simulink model "FOCandPMSM_plant"  (R2022b)
settings: Solver=FixedStepAuto  StartTime=0.0  StopTime=0.25  RelTol=1e-3  EnableMultiTasking=on
PreLoadFcn:
  | Ts = 1e-4;
  | Tcpu = 50e-6; %Controller sample time
  | 
  | % PMSM parameters
  | PM = 0.03; % Permanent magnet flux linkage
  | Ld = 2e-4;  % d-axis inductance
  | Lq = 2e-4;  % q-axis inductance
  | L0 = 2e-4;  % 0-axis inductance
  | Rs = 0.013; % Stator resistance
  | N = 6; % Number of pole pairs
  | J = 0.2; % Moment of inertia
  | 
  | % encoder parameters
  | numSlits = 2000; % number of slits
  | pulseSigOffset = 0; % index pulse signal offset
  | shaftInitPos = 0; % motor shaft initial position
  | 
  | % DAC parameters
  | gain = 0.1;
  | bias = 0;
  | 
  | % circuit parameters
  | Vdc = 48;
  | 
  | % real-time parameters
  | ts_FPGA_clk = 5e-9;
  | ts_FPGA_mdl = 1e-6;
  | 
  | % Real-time processor or embedded controller
  | RTorTTL = 1; % 1: Real-time processor,    0: embedded controller
  | 
  | % sample times
  | f_base = 200e6;
  | PWM_frequency = 20e3;
  | ts_FPGA_clk = 1/f_base;
  | ts_FPGA_mdl =1e-6;
values from neighbouring files (symbols this model uses):
  inverter = mcb_updateInverterParameters(pmsm,inverter,target)    [embedded_sim_codegen_data.m]
  pmsm = mcb_SetPMSMMotorParameters('Teknic2310P')    [embedded_sim_codegen_data.m]
  PU_System = mcb_SetPUSystem(pmsm,inverter)    [embedded_sim_codegen_data.m]
  SpeedRef = 1    [PMSM_HIL_Param.m]
  T_cpu = T_pwm    (= 5e-05)    [embedded_sim_codegen_data.m]
  Tsw = 1/f_sw    [PMSM_HIL_Param.m]
libraries: simulink x5, hdlsllib x3, mcbhdlplantlib x2, slrtencoderlib x2, slrtresolverlib x2, mcbpositiondecoderlib x2, slrthdlutillib x1, slrt2levelinverterlib x1, mcbcontrolslib x1
settings Model: Creator=chrisz  LastModifiedBy=chrisz
settings SolverCC: AutoInsertRateTranBlk=on
settings OptimizationCC: BlockReduction=off  ConditionallyExecuteInputs=off  DefaultParameterBehavior=Inlined
settings DebuggingCC: AlgebraicLoopMsg=error  SingleTaskRateTransMsg=error
settings HardwareCC: ProdBitPerPointer=32  ProdBitPerSizeT=32  ProdBitPerPtrDiffT=32  ProdLargestAtomicFloat=None  ProdIntDivRoundTo=Undefined  ProdEndianess=Unspecified  ProdWordSize=32  ProdHWDeviceType=ASIC/FPGA->ASIC/FPGA  TargetBitPerPointer=64  TargetBitPerSizeT=64  TargetBitPerPtrDiffT=64  TargetLongLongMode=on  TargetIntDivRoundTo=Zero  TargetEndianess=LittleEndian  TargetWordSize=64  TargetHWDeviceType=Custom Processor->MATLAB Host Computer  ProdEqTarget=off
settings ModelReferenceCC: EnableRefExpFcnMdlSchedulingChecks=on

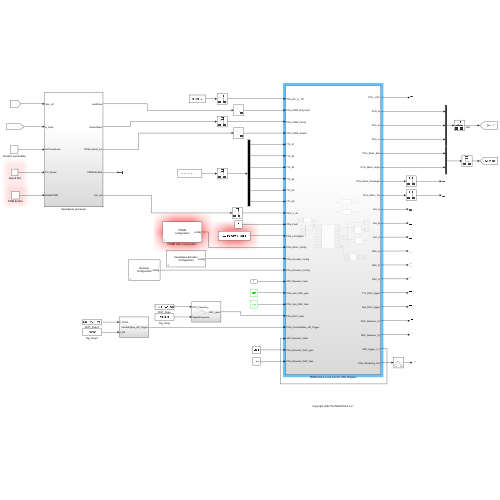
[thumbnail: Simulink's stored preview of the top-level diagram]
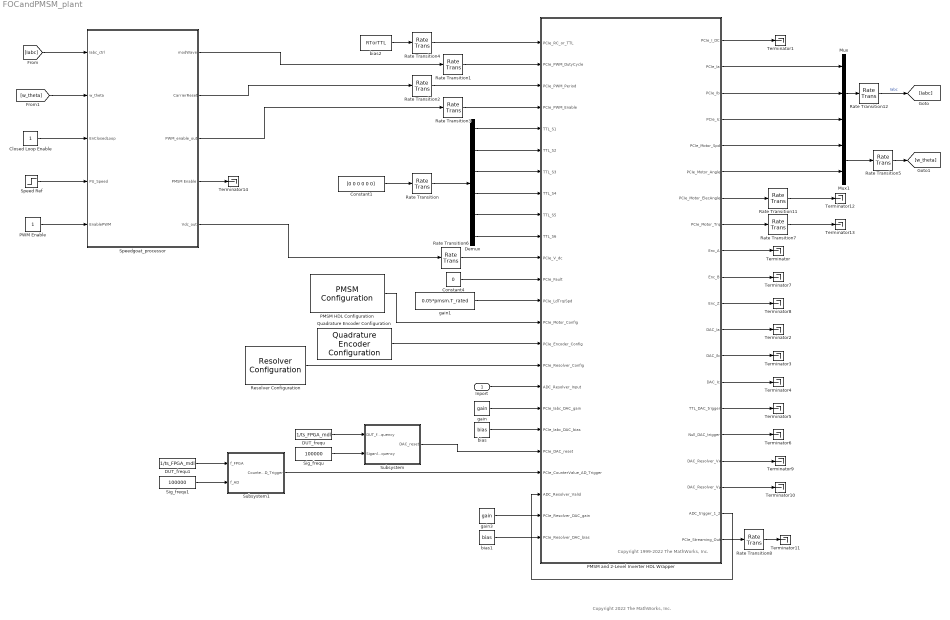
== system FOCandPMSM_plant ==
  note: Copyright 1999-2022 The MathWorks, Inc.
  note: Copyright 2022 The MathWorks, Inc.
  Inport : Inport  OutDataTypeStr=int16
  Closed Loop Enable : Constant  OutDataTypeStr=Inherit: Inherit via back propagation  SampleTime=-1
  Constant1 : Constant  Value=[0 0 0 0 0 0]  OutDataTypeStr=boolean  SampleTime=-1
  Constant4 : Constant  Value=0  OutDataTypeStr=uint32  SampleTime=ts_FPGA_mdl
  DUT_frequ : Constant  Value=1/ts_FPGA_mdl  SampleTime=ts_FPGA_mdl
  DUT_frequ1 : Constant  Value=1/ts_FPGA_mdl  SampleTime=ts_FPGA_mdl
  Demux : Demux  Outputs=6
  Mux : Mux  Inputs=3
  Mux1 : Mux  Inputs=2
  PMSM HDL Configuration : mcbhdlplantlib/PMSM Configuration  portConfig=Torque  Trq_N_mode=0  Ts=ts_FPGA_mdl  Pp=pmsm.p  Rs=pmsm.Rs  Ld=pmsm.Ld  Lq=pmsm.Lq  lambda_pm=pmsm.FluxPM  J=pmsm.J  B=0  f=0
      settings: LibrarySourceBlock=mcbhdllib/Electrical Systems/Motors/PMSM Configuration
  PMSM and 2-Level Inverter HDL Wrapper : Subsystem
  PWM Enable : Constant  OutDataTypeStr=Inherit: Inherit via back propagation  SampleTime=T_cpu
  Quadrature Encoder Configuration : slrtencoderlib/Quadrature Encoder Configuration  NPulses=2000  zOffset=0  Ts=ts_FPGA_mdl
  Rate Transition : RateTransition  OutPortSampleTime=ts_FPGA_clk
  Rate Transition{1..4,6} (5 alike) : RateTransition  OutPortSampleTime=ts_FPGA_mdl
  Rate Transition{5,7..8,11..12} (5 alike) : RateTransition  OutPortSampleTime=Tcpu
  Resolver Configuration : slrtresolverlib/Resolver Configuration  Ts=ts_FPGA_mdl  R=0.5  N=1  ADCrefV=5  ADCbits=16  totalADCCounts=65536
  Sig_frequ : Constant  Value=100000  VectorParams1D=off  SampleTime=ts_FPGA_mdl
  Sig_frequ1 : Constant  Value=100000  VectorParams1D=off  SampleTime=ts_FPGA_mdl
  Speed Ref : Step  Time=0.25  Before=1500/PU_System.N_base  After=SpeedRef  OutDataTypeStr=dataType  SampleTime=T_cpu
  Speedgoat_processor : Subsystem
  Subsystem : Subsystem
  Subsystem1 : Subsystem
  Terminator{,1..14} (15 alike) : Terminator
  bias : Constant  Value=bias  OutDataTypeStr=single  SampleTime=ts_FPGA_mdl
  bias1 : Constant  Value=bias  OutDataTypeStr=single  SampleTime=ts_FPGA_mdl
  bias2 : Constant  Value=RTorTTL  OutDataTypeStr=single  SampleTime=ts_FPGA_mdl
  gain : Constant  Value=gain  OutDataTypeStr=single  SampleTime=ts_FPGA_mdl
  gain1 : Constant  Value=0.05*pmsm.T_rated  OutDataTypeStr=single  SampleTime=ts_FPGA_mdl
  gain3 : Constant  Value=gain  OutDataTypeStr=single  SampleTime=ts_FPGA_mdl
  wires:
  PMSM and 2-Level Inverter HDL Wrapper/9(Enc_A) -> Terminator/1
  Rate Transition7/1 -> Terminator13/1
  PMSM and 2-Level Inverter HDL Wrapper/12(DAC_Ia) -> Terminator2/1
  PMSM and 2-Level Inverter HDL Wrapper/1(PCIe_I_DC) -> Terminator1/1
  PMSM and 2-Level Inverter HDL Wrapper/10(Enc_B) -> Terminator7/1
  PMSM and 2-Level Inverter HDL Wrapper/14(DAC_Ic) -> Terminator4/1
  PMSM and 2-Level Inverter HDL Wrapper/15(TTL_DAC_trigger) -> Terminator5/1
  PMSM and 2-Level Inverter HDL Wrapper/13(DAC_Ib) -> Terminator3/1
  PMSM and 2-Level Inverter HDL Wrapper/16(Null_DAC_trigger) -> Terminator6/1
  PMSM and 2-Level Inverter HDL Wrapper/5(PCIe_Motor_Spd) -> Mux1/1
  PMSM and 2-Level Inverter HDL Wrapper/6(PCIe_Motor_Angle) -> Mux1/2
  PMSM and 2-Level Inverter HDL Wrapper/8(PCIe_Motor_Trq) -> Rate Transition7/1
  PMSM and 2-Level Inverter HDL Wrapper/11(Enc_Z) -> Terminator8/1
  PMSM and 2-Level Inverter HDL Wrapper/17(DAC_Resolver_Vx) -> Terminator9/1
  PMSM and 2-Level Inverter HDL Wrapper/18(DAC_Resolver_Vy) -> Terminator10/1
  Rate Transition11/1 -> Terminator12/1
  PMSM and 2-Level Inverter HDL Wrapper/7(PCIe_Motor_ElecAngle) -> Rate Transition11/1
  Speedgoat_processor/4(PMSM Enable) -> Terminator14/1
  Demux/4 -> PMSM and 2-Level Inverter HDL Wrapper/8(TTL_S4)
  gain3/1 -> PMSM and 2-Level Inverter HDL Wrapper/23(PCIe_Resolver_DAC_gain)
  Subsystem/1(DAC_reset) -> PMSM and 2-Level Inverter HDL Wrapper/20(PCIe_DAC_reset)
  Rate Transition1/1 -> PMSM and 2-Level Inverter HDL Wrapper/2(PCIe_PWM_DutyCycle)
  Demux/2 -> PMSM and 2-Level Inverter HDL Wrapper/6(TTL_S2)
  Subsystem1/1(CounterValue_AD_Trigger) -> PMSM and 2-Level Inverter HDL Wrapper/21(PCIe_CounterValue_AD_Trigger)
  Demux/1 -> PMSM and 2-Level Inverter HDL Wrapper/5(TTL_S1)
  bias/1 -> PMSM and 2-Level Inverter HDL Wrapper/19(PCIe_Iabc_DAC_bias)
  Rate Transition4/1 -> PMSM and 2-Level Inverter HDL Wrapper/1(PCIe_RC_or_TTL)
  bias1/1 -> PMSM and 2-Level Inverter HDL Wrapper/24(PCIe_Resolver_DAC_bias)
  gain/1 -> PMSM and 2-Level Inverter HDL Wrapper/18(PCIe_Iabc_DAC_gain)
  Constant4/1 -> PMSM and 2-Level Inverter HDL Wrapper/12(PCIe_Fault)
  Rate Transition3/1 -> PMSM and 2-Level Inverter HDL Wrapper/4(PCIe_PWM_Enable)
  Rate Transition2/1 -> PMSM and 2-Level Inverter HDL Wrapper/3(PCIe_PWM_Period)
  Demux/3 -> PMSM and 2-Level Inverter HDL Wrapper/7(TTL_S3)
  PMSM HDL Configuration/1 -> PMSM and 2-Level Inverter HDL Wrapper/14(PCIe_Motor_Config)
  gain1/1 -> PMSM and 2-Level Inverter HDL Wrapper/13(PCIe_LdTrq/Spd)
  Resolver Configuration/1 -> PMSM and 2-Level Inverter HDL Wrapper/16(PCIe_Resolver_Config)
  PWM Enable/1 -> Speedgoat_processor/5(EnablePWM)
  Inport/1 -> PMSM and 2-Level Inverter HDL Wrapper/17(ADC_Resolver_Input)
  Speedgoat_processor/3(PWM_enable_out) -> Rate Transition3/1
  [Iabc] -> Speedgoat_processor/1(Iabc_ctrl)
  DUT_frequ1/1 -> Subsystem1/1(f_FPGA)
  DUT_frequ/1 -> Subsystem/1(DUT_frequency)
  Speed Ref/1 -> Speedgoat_processor/4(PU_Speed)
  Speedgoat_processor/2(CarrierReset) -> Rate Transition2/1
  bias2/1 -> Rate Transition4/1
  Closed Loop Enable/1 -> Speedgoat_processor/3(EnClosedLoop)
  Sig_frequ1/1 -> Subsystem1/2(f_AD)
  Sig_frequ/1 -> Subsystem/2(SiganlFrequency)
  Speedgoat_processor/1(modWave) -> Rate Transition1/1
  Constant1/1 -> Rate Transition/1
  Demux/6 -> PMSM and 2-Level Inverter HDL Wrapper/10(TTL_S6)
  Quadrature Encoder Configuration/1 -> PMSM and 2-Level Inverter HDL Wrapper/15(PCIe_Encoder_Config)
  Demux/5 -> PMSM and 2-Level Inverter HDL Wrapper/9(TTL_S5)
  [w_theta] -> Speedgoat_processor/2(w_theta)
  Rate Transition/1 -> Demux/1
  PMSM and 2-Level Inverter HDL Wrapper/19(ADC_trigger_1_2) -> PMSM and 2-Level Inverter HDL Wrapper/22(ADC_Resolver_Valid)
  Mux/1 -> Rate Transition12/1
  Rate Transition5/1 -> [w_theta]
  Mux1/1 -> Rate Transition5/1
  Speedgoat_processor/5(Vdc_out) -> Rate Transition6/1
  Rate Transition6/1 -> PMSM and 2-Level Inverter HDL Wrapper/11(PCIe_V_dc)
  PMSM and 2-Level Inverter HDL Wrapper/2(PCIe_Ia) -> Mux/1
  PMSM and 2-Level Inverter HDL Wrapper/3(PCIe_Ib) -> Mux/2
  PMSM and 2-Level Inverter HDL Wrapper/4(PCIe_Ic) -> Mux/3
  Rate Transition12/1 -> [Iabc]  "Iabc"
  PMSM and 2-Level Inverter HDL Wrapper/20(PCIe_Streaming_Out) -> Rate Transition8/1
  Rate Transition8/1 -> Terminator11/1

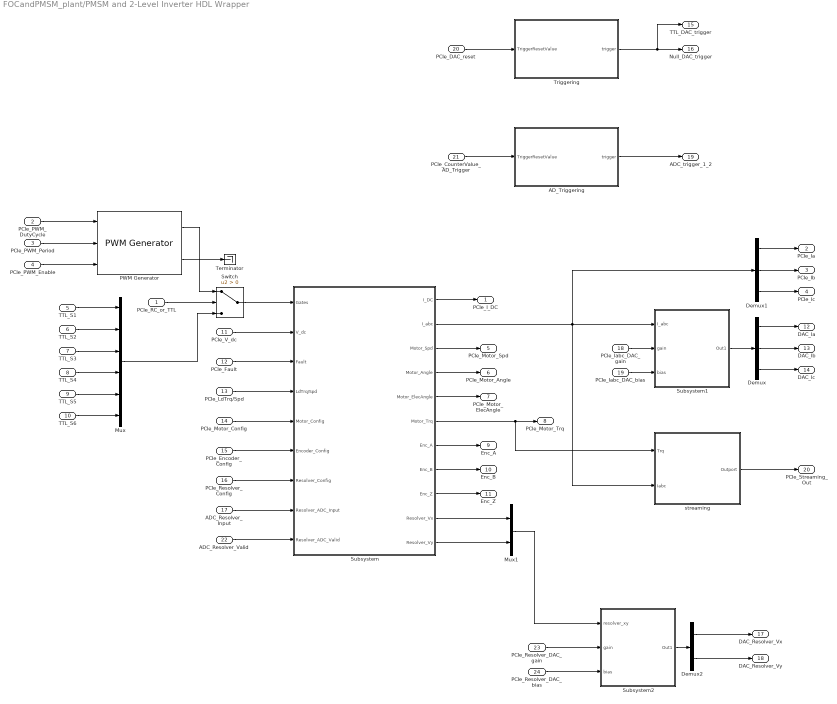
== system FOCandPMSM_plant/PMSM and 2-Level Inverter HDL Wrapper ==
  PCIe_RC_or_TTL : Inport
  PCIe_PWM_DutyCycle : Inport  Port=2
  PCIe_PWM_Period : Inport  Port=3
  PCIe_PWM_Enable : Inport  Port=4
  TTL_S1 : Inport  Port=5
  TTL_S2 : Inport  Port=6
  TTL_S3 : Inport  Port=7
  TTL_S4 : Inport  Port=8
  TTL_S5 : Inport  Port=9
  TTL_S6 : Inport  Port=10
  PCIe_V_dc : Inport  Port=11
  PCIe_Fault : Inport  Port=12
  PCIe_LdTrq/Spd : Inport  Port=13
  PCIe_Motor_Config : Inport  Port=14
  PCIe_Encoder_Config : Inport  Port=15
  PCIe_Resolver_Config : Inport  Port=16
  ADC_Resolver_Input : Inport  Port=17
  PCIe_Iabc_DAC_gain : Inport  Port=18
  PCIe_Iabc_DAC_bias : Inport  Port=19
  PCIe_DAC_reset : Inport  Port=20
  PCIe_CounterValue_AD_Trigger : Inport  Port=21  OutDataTypeStr=uint32
  ADC_Resolver_Valid : Inport  Port=22
  PCIe_Resolver_DAC_gain : Inport  Port=23
  PCIe_Resolver_DAC_bias : Inport  Port=24
  AD_Triggering : Subsystem
  Demux : Demux  Outputs=3
  Demux1 : Demux  Outputs=3
  Demux2 : Demux  Outputs=2
  Mux : Mux  Inputs=6
  Mux1 : Mux  Inputs=2
  PWM Generator : slrthdlutillib/PWM Generator
  Subsystem : Subsystem
  Subsystem1 : Subsystem
  Subsystem2 : Subsystem
  Switch : Switch  Criteria=u2 > Threshold  SaturateOnIntegerOverflow=off  InputSameDT=off
  Terminator : Terminator
  Triggering : Subsystem
  streaming : Subsystem
  PCIe_I_DC : Outport
  PCIe_Ia : Outport  Port=2
  PCIe_Ib : Outport  Port=3
  PCIe_Ic : Outport  Port=4
  PCIe_Motor_Spd : Outport  Port=5
  PCIe_Motor_Angle : Outport  Port=6
  PCIe_Motor_ElecAngle : Outport  Port=7
  PCIe_Motor_Trq : Outport  Port=8
  Enc_A : Outport  Port=9
  Enc_B : Outport  Port=10
  Enc_Z : Outport  Port=11
  DAC_Ia : Outport  Port=12
  DAC_Ib : Outport  Port=13
  DAC_Ic : Outport  Port=14
  TTL_DAC_trigger : Outport  Port=15
  Null_DAC_trigger : Outport  Port=16
  DAC_Resolver_Vx : Outport  Port=17
  DAC_Resolver_Vy : Outport  Port=18
  ADC_trigger_1_2 : Outport  Port=19  OutDataTypeStr=boolean
  PCIe_Streaming_Out : Outport  Port=20
  wires:
  Subsystem/7(Enc_A) -> Enc_A/1
  TTL_S2/1 -> Mux/2
  Demux1/1 -> PCIe_Ia/1
  PCIe_PWM_DutyCycle/1 -> PWM Generator/1
  TTL_S5/1 -> Mux/5
  Subsystem/2(I_abc) -> Demux1/1, streaming/2(Iabc), Subsystem1/1(I_abc)
  Subsystem/6(Motor_Trq) -> streaming/1(Trq), PCIe_Motor_Trq/1
  Subsystem/4(Motor_Angle) -> PCIe_Motor_Angle/1
  Subsystem/1(I_DC) -> PCIe_I_DC/1
  PCIe_Encoder_Config/1 -> Subsystem/6(Encoder_Config)
  PCIe_Iabc_DAC_bias/1 -> Subsystem1/3(bias)
  Subsystem/3(Motor_Spd) -> PCIe_Motor_Spd/1
  Subsystem/8(Enc_B) -> Enc_B/1
  PCIe_V_dc/1 -> Subsystem/2(V_dc)
  PWM Generator/1 -> Switch/1
  Triggering/1(trigger) -> Null_DAC_trigger/1, TTL_DAC_trigger/1
  TTL_S6/1 -> Mux/6
  Subsystem/9(Enc_Z) -> Enc_Z/1
  PCIe_LdTrq/Spd/1 -> Subsystem/4(LdTrq/Spd)
  TTL_S1/1 -> Mux/1
  Demux1/3 -> PCIe_Ic/1
  Demux1/2 -> PCIe_Ib/1
  PCIe_RC_or_TTL/1 -> Switch/2
  PCIe_Motor_Config/1 -> Subsystem/5(Motor_Config)
  Demux/1 -> DAC_Ia/1
  Mux/1 -> Switch/3
  PCIe_PWM_Period/1 -> PWM Generator/2
  TTL_S4/1 -> Mux/4
  PCIe_Fault/1 -> Subsystem/3(Fault)
  PCIe_DAC_reset/1 -> Triggering/1(TriggerResetValue)
  PCIe_Iabc_DAC_gain/1 -> Subsystem1/2(gain)
  PCIe_PWM_Enable/1 -> PWM Generator/3
  Demux/2 -> DAC_Ib/1
  Switch/1 -> Subsystem/1(Gates)
  Subsystem1/1(Out1) -> Demux/1
  TTL_S3/1 -> Mux/3
  Demux/3 -> DAC_Ic/1
  PCIe_Resolver_Config/1 -> Subsystem/7(Resolver_Config)
  ADC_Resolver_Input/1 -> Subsystem/8(Resolver_ADC_Input)
  PCIe_CounterValue_AD_Trigger/1 -> AD_Triggering/1(TriggerResetValue)
  AD_Triggering/1(trigger) -> ADC_trigger_1_2/1
  ADC_Resolver_Valid/1 -> Subsystem/9(Resolver_ADC_Valid)
  Subsystem/5(Motor_ElecAngle) -> PCIe_Motor_ElecAngle/1
  streaming/1(Outport) -> PCIe_Streaming_Out/1
  Subsystem/10(Resolver_Vx) -> Mux1/1
  Subsystem/11(Resolver_Vy) -> Mux1/2
  Mux1/1 -> Subsystem2/1(resolver_xy)
  PCIe_Resolver_DAC_gain/1 -> Subsystem2/2(gain)
  PCIe_Resolver_DAC_bias/1 -> Subsystem2/3(bias)
  Subsystem2/1(Out1) -> Demux2/1
  Demux2/1 -> DAC_Resolver_Vx/1
  Demux2/2 -> DAC_Resolver_Vy/1
  PWM Generator/2 -> Terminator/1

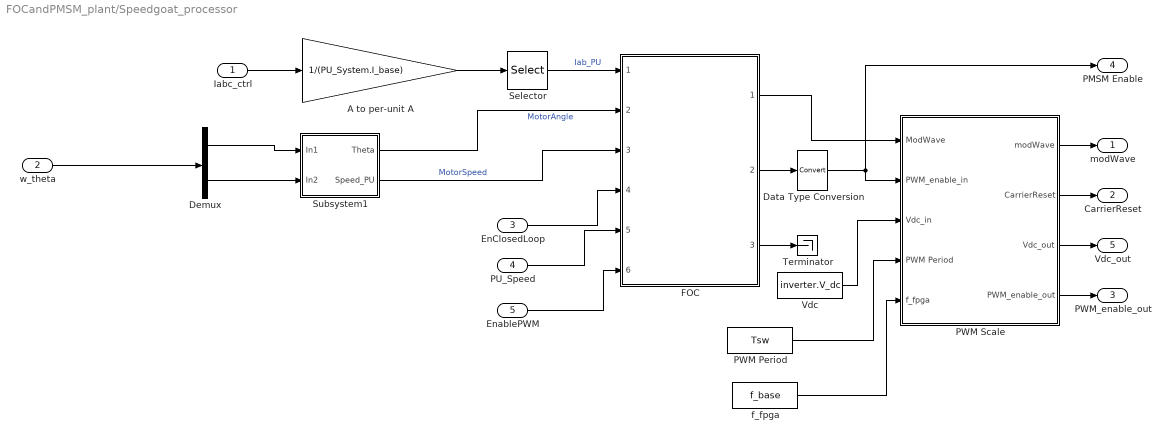
== system FOCandPMSM_plant/Speedgoat_processor ==
  Iabc_ctrl : Inport
  w_theta : Inport  Port=2
  EnClosedLoop : Inport  Port=3
  PU_Speed : Inport  Port=4
  EnablePWM : Inport  Port=5
  A to per-unit A : Gain  Gain=1/(PU_System.I_base)
  Data Type Conversion : DataTypeConversion  SaturateOnIntegerOverflow=off  RndMeth=Floor
  Demux : Demux  Outputs=2
  FOC : Subsystem  ReferencedSubsystem=Field_Oriented_Control  AxisAlignment=D-axis
  PWM Period : Constant  Value=Tsw  SampleTime=-1
  PWM Scale : Subsystem
  Selector : Selector  InputPortWidth=3  IndexOptions=Index vector (dialog)  Indices=[1 2]  OutputSizes=1
  Subsystem1 : Subsystem
  Terminator : Terminator
  Vdc : Constant  Value=inverter.V_dc  OutDataTypeStr=single  SampleTime=T_cpu
  f_fpga : Constant  Value=f_base  SampleTime=-1
  modWave : Outport
  CarrierReset : Outport  Port=2
  PWM_enable_out : Outport  Port=3
  PMSM Enable : Outport  Port=4
  Vdc_out : Outport  Port=5
  wires:
  Data Type Conversion/1 -> PMSM Enable/1, PWM Scale/2(PWM_enable_in)
  f_fpga/1 -> PWM Scale/5(f_fpga)
  PWM Period/1 -> PWM Scale/4(PWM Period)
  Vdc/1 -> PWM Scale/3(Vdc_in)
  Subsystem1/1(Theta) -> FOC/2  "MotorAngle"
  FOC/3 -> Terminator/1
  FOC/2 -> Data Type Conversion/1
  Demux/2 -> Subsystem1/2(In2)
  Subsystem1/2(Speed_PU) -> FOC/3  "MotorSpeed"
  Iabc_ctrl/1 -> A to per-unit A/1
  Demux/1 -> Subsystem1/1(In1)
  A to per-unit A/1 -> Selector/1
  FOC/1 -> PWM Scale/1(ModWave)
  PWM Scale/3(Vdc_out) -> Vdc_out/1
  Selector/1 -> FOC/1  "Iab_PU"
  w_theta/1 -> Demux/1
  EnablePWM/1 -> FOC/6
  PU_Speed/1 -> FOC/5
  PWM Scale/2(CarrierReset) -> CarrierReset/1
  PWM Scale/4(PWM_enable_out) -> PWM_enable_out/1
  EnClosedLoop/1 -> FOC/4
  PWM Scale/1(modWave) -> modWave/1

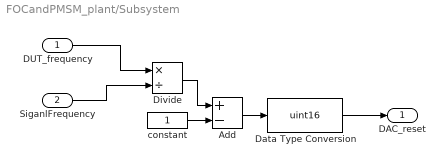
== system FOCandPMSM_plant/Subsystem ==
  DUT_frequency : Inport
  SiganlFrequency : Inport  Port=2
  Add : Sum  Inputs=+-
  Data Type Conversion : DataTypeConversion  OutDataTypeStr=uint16  SaturateOnIntegerOverflow=off  RndMeth=Floor
  Divide : Product  Inputs=*/
  constant : Constant  VectorParams1D=off  SampleTime=-1
  DAC_reset : Outport
  wires:
  SiganlFrequency/1 -> Divide/2
  Add/1 -> Data Type Conversion/1
  Divide/1 -> Add/1
  Data Type Conversion/1 -> DAC_reset/1
  constant/1 -> Add/2
  DUT_frequency/1 -> Divide/1

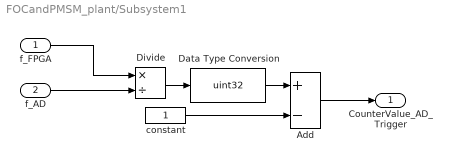
== system FOCandPMSM_plant/Subsystem1 ==
  f_FPGA : Inport
  f_AD : Inport  Port=2
  Add : Sum  Inputs=+-  AccumDataTypeStr=uint32
  Data Type Conversion : DataTypeConversion  OutDataTypeStr=uint32  SaturateOnIntegerOverflow=off  RndMeth=Floor
  Divide : Product  Inputs=*/
  constant : Constant  VectorParams1D=off  OutDataTypeStr=uint32  SampleTime=-1
  CounterValue_AD_Trigger : Outport
  wires:
  Add/1 -> CounterValue_AD_Trigger/1
  constant/1 -> Add/2
  Data Type Conversion/1 -> Add/1
  Divide/1 -> Data Type Conversion/1
  f_FPGA/1 -> Divide/1
  f_AD/1 -> Divide/2

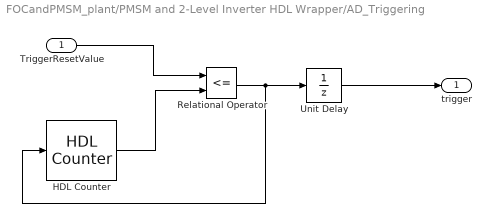
== system FOCandPMSM_plant/PMSM and 2-Level Inverter HDL Wrapper/AD_Triggering ==
  TriggerResetValue : Inport
  HDL Counter : hdlsllib/Sources/HDL Counter  CountType=Free running  CountInit=0  CountStep=1  CountMax=25  CountFromType=Initial value  CountFrom=0  CountResetPort=on  CountLoadPort=off  CountEnbPort=off  CountDirPort=off  CountHitOutputPort=off  CountDataType=Unsigned  CountWordLen=32  CountFracLen=0  CountSampTime=1
  Relational Operator : RelationalOperator  Operator=<=  OutDataTypeStr=boolean  InputSameDT=off
  Unit Delay : UnitDelay  SampleTime=-1  HasFrameUpgradeWarning=on
  trigger : Outport
  wires:
  TriggerResetValue/1 -> Relational Operator/1
  HDL Counter/1 -> Relational Operator/2
  Relational Operator/1 -> HDL Counter/1, Unit Delay/1
  Unit Delay/1 -> trigger/1

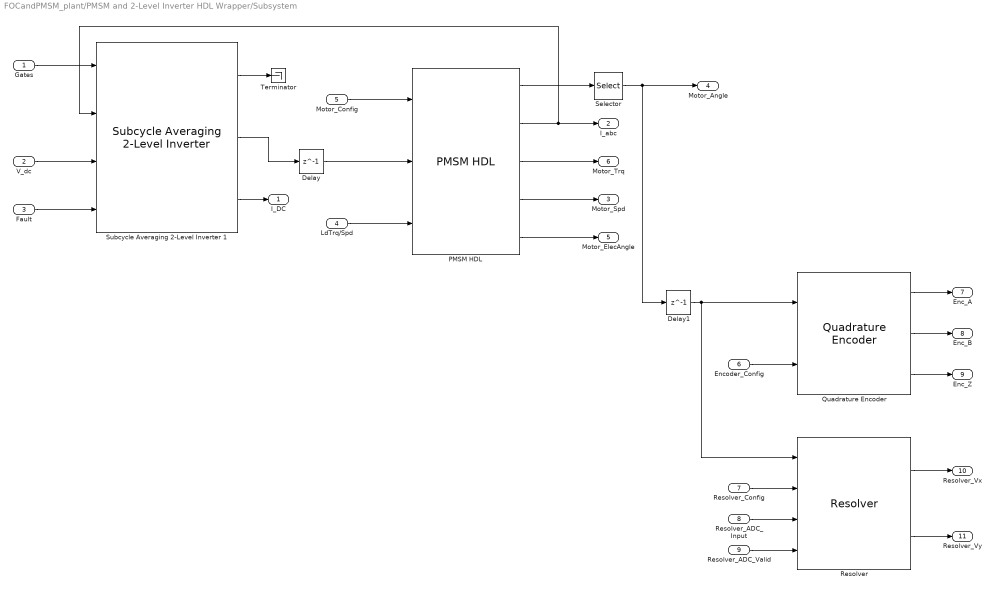
== system FOCandPMSM_plant/PMSM and 2-Level Inverter HDL Wrapper/Subsystem ==
  Gates : Inport
  V_dc : Inport  Port=2
  Fault : Inport  Port=3
  LdTrq/Spd : Inport  Port=4
  Motor_Config : Inport  Port=5
  Encoder_Config : Inport  Port=6
  Resolver_Config : Inport  Port=7
  Resolver_ADC_Input : Inport  Port=8
  Resolver_ADC_Valid : Inport  Port=9
  Delay : Delay  DelayLength=1
  Delay1 : Delay  DelayLength=1
  PMSM HDL : mcbhdlplantlib/PMSM HDL  VariantControl=pmsmVariant==pmsmEnum.TorqueInput  Ts=1e-6
  Quadrature Encoder : slrtencoderlib/Quadrature Encoder
  Resolver : slrtresolverlib/Resolver  Ts=ts_FPGA_mdl
  Selector : Selector  InputPortWidth=14  IndexOptions=Index vector (dialog)  Indices=[10]  OutputSizes=1
  Subcycle Averaging 2-Level Inverter 1 : slrt2levelinverterlib/Subcycle Averaging 2-Level Inverter   rSwitch=0.001  vfSwitch=0.1  rDiode=0.001  vfDiode=0.8  rSnub=100  ts_Model=ts_FPGA_mdl  ts_FPGA=ts_FPGA_clk
  Terminator : Terminator
  I_DC : Outport
  I_abc : Outport  Port=2
  Motor_Spd : Outport  Port=3
  Motor_Angle : Outport  Port=4
  Motor_ElecAngle : Outport  Port=5
  Motor_Trq : Outport  Port=6
  Enc_A : Outport  Port=7
  Enc_B : Outport  Port=8
  Enc_Z : Outport  Port=9
  Resolver_Vx : Outport  Port=10
  Resolver_Vy : Outport  Port=11
  wires:
  Motor_Config/1 -> PMSM HDL/1
  Subcycle Averaging 2-Level Inverter 1/3 -> I_DC/1
  V_dc/1 -> Subcycle Averaging 2-Level Inverter 1/3
  PMSM HDL/2 -> Subcycle Averaging 2-Level Inverter 1/2, I_abc/1
  Quadrature Encoder/2 -> Enc_B/1
  Fault/1 -> Subcycle Averaging 2-Level Inverter 1/4
  Quadrature Encoder/1 -> Enc_A/1
  PMSM HDL/3 -> Motor_Trq/1
  LdTrq/Spd/1 -> PMSM HDL/3
  Quadrature Encoder/3 -> Enc_Z/1
  PMSM HDL/4 -> Motor_Spd/1
  Encoder_Config/1 -> Quadrature Encoder/2
  Gates/1 -> Subcycle Averaging 2-Level Inverter 1/1
  Resolver_Config/1 -> Resolver/2
  Resolver_ADC_Input/1 -> Resolver/3
  Resolver/1 -> Resolver_Vx/1
  Resolver/2 -> Resolver_Vy/1
  Resolver_ADC_Valid/1 -> Resolver/4
  Subcycle Averaging 2-Level Inverter 1/1 -> Terminator/1
  PMSM HDL/1 -> Selector/1
  PMSM HDL/5 -> Motor_ElecAngle/1
  Subcycle Averaging 2-Level Inverter 1/2 -> Delay/1
  Delay/1 -> PMSM HDL/2
  Selector/1 -> Delay1/1, Motor_Angle/1
  Delay1/1 -> Resolver/1, Quadrature Encoder/1

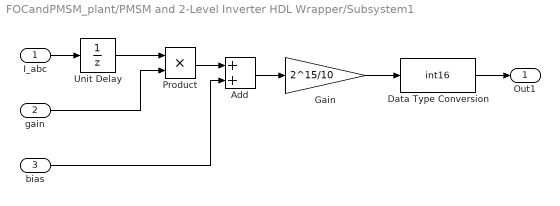
== system FOCandPMSM_plant/PMSM and 2-Level Inverter HDL Wrapper/Subsystem1 ==
  I_abc : Inport
  gain : Inport  Port=2
  bias : Inport  Port=3
  Add : Sum
  Data Type Conversion : DataTypeConversion  OutDataTypeStr=int16  SaturateOnIntegerOverflow=off  RndMeth=Floor
  Gain : Gain  Gain=2^15/10
  Product : Product
  Unit Delay : UnitDelay  SampleTime=-1  HasFrameUpgradeWarning=on
  Out1 : Outport
  wires:
  I_abc/1 -> Unit Delay/1
  Unit Delay/1 -> Product/1
  gain/1 -> Product/2
  Product/1 -> Add/1
  bias/1 -> Add/2
  Add/1 -> Gain/1
  Gain/1 -> Data Type Conversion/1
  Data Type Conversion/1 -> Out1/1

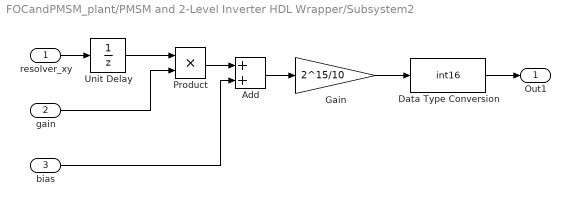
== system FOCandPMSM_plant/PMSM and 2-Level Inverter HDL Wrapper/Subsystem2 ==
  resolver_xy : Inport
  gain : Inport  Port=2
  bias : Inport  Port=3
  Add : Sum
  Data Type Conversion : DataTypeConversion  OutDataTypeStr=int16  SaturateOnIntegerOverflow=off  RndMeth=Floor
  Gain : Gain  Gain=2^15/10
  Product : Product
  Unit Delay : UnitDelay  SampleTime=-1  HasFrameUpgradeWarning=on
  Out1 : Outport
  wires:
  resolver_xy/1 -> Unit Delay/1
  Unit Delay/1 -> Product/1
  gain/1 -> Product/2
  Product/1 -> Add/1
  bias/1 -> Add/2
  Add/1 -> Gain/1
  Gain/1 -> Data Type Conversion/1
  Data Type Conversion/1 -> Out1/1

== system FOCandPMSM_plant/PMSM and 2-Level Inverter HDL Wrapper/Triggering ==
  TriggerResetValue : Inport
  HDL Counter : hdlsllib/Sources/HDL Counter  CountType=Free running  CountInit=0  CountStep=1  CountMax=25  CountFromType=Initial value  CountFrom=0  CountResetPort=on  CountLoadPort=off  CountEnbPort=off  CountDirPort=off  CountHitOutputPort=off  CountDataType=Unsigned  CountWordLen=16  CountFracLen=0  CountSampTime=1
  Relational Operator : RelationalOperator  Operator===  OutDataTypeStr=boolean  InputSameDT=off
  Unit Delay : UnitDelay  SampleTime=-1  HasFrameUpgradeWarning=on
  trigger : Outport
  wires:
  TriggerResetValue/1 -> Relational Operator/1
  HDL Counter/1 -> Relational Operator/2
  Relational Operator/1 -> HDL Counter/1, Unit Delay/1
  Unit Delay/1 -> trigger/1

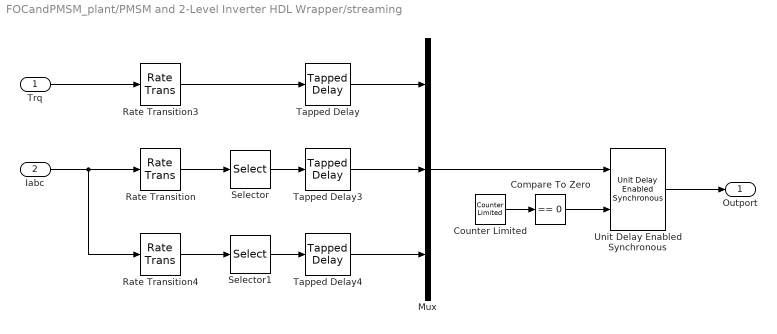
== system FOCandPMSM_plant/PMSM and 2-Level Inverter HDL Wrapper/streaming ==
  Trq : Inport
  Iabc : Inport  Port=2
  Compare To Zero : simulink/Logic and Bit Operations/Compare To Zero  relop===  OutDataTypeStr=boolean
  Counter Limited : simulink/Sources/Counter Limited  uplimit=49  tsamp=Tcpu
  Mux : Mux  Inputs=3
  Rate Transition : RateTransition
  Rate Transition3 : RateTransition
  Rate Transition4 : RateTransition
  Selector : Selector  InputPortWidth=3  IndexOptions=Index vector (dialog)  Indices=[1]  OutputSizes=1
  Selector1 : Selector  InputPortWidth=3  IndexOptions=Index vector (dialog)  Indices=[2]  OutputSizes=1
  Tapped Delay : simulink/Discrete/Tapped Delay  vinit=0.0  samptime=Tcpu  NumDelays=50  DelayOrder=Oldest  includeCurrent=off
  Tapped Delay3 : simulink/Discrete/Tapped Delay  vinit=0.0  samptime=Tcpu  NumDelays=50  DelayOrder=Oldest  includeCurrent=off
  Tapped Delay4 : simulink/Discrete/Tapped Delay  vinit=0.0  samptime=Tcpu  NumDelays=50  DelayOrder=Oldest  includeCurrent=off
  Unit Delay Enabled Synchronous : hdlsllib/Discrete/Unit Delay Enabled Synchronous  InitialCondition=0.0  SampleTime=-1
  Outport : Outport
  wires:
  Iabc/1 -> Rate Transition4/1, Rate Transition/1
  Trq/1 -> Rate Transition3/1
  Rate Transition3/1 -> Tapped Delay/1
  Rate Transition/1 -> Selector/1
  Rate Transition4/1 -> Selector1/1
  Selector/1 -> Tapped Delay3/1
  Selector1/1 -> Tapped Delay4/1
  Tapped Delay/1 -> Mux/1
  Tapped Delay3/1 -> Mux/2
  Tapped Delay4/1 -> Mux/3
  Mux/1 -> Unit Delay Enabled Synchronous/1
  Counter Limited/1 -> Compare To Zero/1
  Compare To Zero/1 -> Unit Delay Enabled Synchronous/2
  Unit Delay Enabled Synchronous/1 -> Outport/1

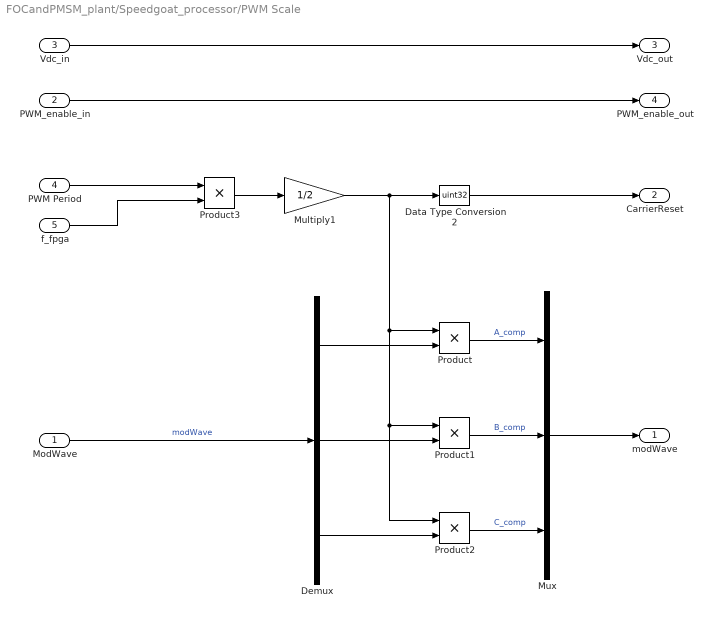
== system FOCandPMSM_plant/Speedgoat_processor/PWM Scale ==
  ModWave : Inport
  PWM_enable_in : Inport  Port=2
  Vdc_in : Inport  Port=3
  PWM Period : Inport  Port=4
  f_fpga : Inport  Port=5
  Data Type Conversion2 : DataTypeConversion  OutDataTypeStr=uint32  SaturateOnIntegerOverflow=off  RndMeth=Floor
  Demux : Demux  Outputs=3
  Multiply1 : Gain  Gain=1/2
  Mux : Mux  Inputs=3
  Product : Product  OutDataTypeStr=uint32
  Product1 : Product  OutDataTypeStr=uint32
  Product2 : Product  OutDataTypeStr=uint32
  Product3 : Product
  modWave : Outport  VectorParamsAs1DForOutWhenUnconnected=off
  CarrierReset : Outport  Port=2  VectorParamsAs1DForOutWhenUnconnected=off
  Vdc_out : Outport  Port=3  VectorParamsAs1DForOutWhenUnconnected=off
  PWM_enable_out : Outport  Port=4  VectorParamsAs1DForOutWhenUnconnected=off
  wires:
  ModWave/1 -> Demux/1  "modWave"
  Multiply1/1 -> Product2/1, Product1/1, Product/1, Data Type Conversion2/1
  PWM Period/1 -> Product3/1
  Data Type Conversion2/1 -> CarrierReset/1
  Demux/1 -> Product/2
  Demux/2 -> Product1/2
  Demux/3 -> Product2/2
  f_fpga/1 -> Product3/2
  Product3/1 -> Multiply1/1
  Product1/1 -> Mux/2  "B_comp"
  Product/1 -> Mux/1  "A_comp"
  Product2/1 -> Mux/3  "C_comp"
  Vdc_in/1 -> Vdc_out/1
  PWM_enable_in/1 -> PWM_enable_out/1
  Mux/1 -> modWave/1

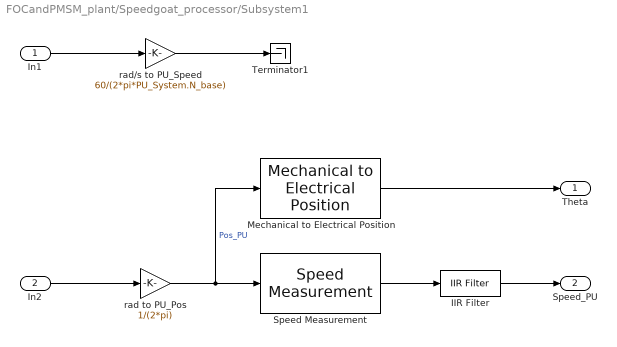
== system FOCandPMSM_plant/Speedgoat_processor/Subsystem1 ==
  In1 : Inport
  In2 : Inport  Port=2
  IIR Filter : mcbcontrolslib/IIR Filter  VariantControl=Low Pass Filter  VariantSelect=Low-pass  Filter_constant=0.01  advancedSettings=off  Ts=50e-6  cutOff_freq=32.1525
  Mechanical to Electrical Position : mcbpositiondecoderlib/Mechanical to Electrical Position  NrPP=pmsm.p  selectedRange=Per unit  MechOfstInputType=Specify via dialog  mechOffsetIn=0  maxAngleIn=1  InputDataType=single  VariantSelect=floating-point
  Speed Measurement : mcbpositiondecoderlib/Speed Measurement  PositionUnit=Per unit  PositionScalingDatatype=uint32  SpeedCalculationMode=Time interval for speed calculation  SampleTimeAsync=T_cpu  MaximumApplicationSpeed=6000  SpeedResolution=5e-6  DelayLength=20  MaximumMeasurableSpeed=29999  MeasurableSpeedResolution=1.397e-05  SpeedUnit=Per unit based on dialog  PerUnitSpeed=PU_System.N_base  SpeedDataType=dataType
  Terminator1 : Terminator
  rad to PU_Pos : Gain  Gain=1/(2*pi)
  rad/s to PU_Speed : Gain  Gain=60/(2*pi*PU_System.N_base)
  Theta : Outport
  Speed_PU : Outport  Port=2
  wires:
  In1/1 -> rad/s to PU_Speed/1
  Speed Measurement/1 -> IIR Filter/1
  In2/1 -> rad to PU_Pos/1
  Mechanical to Electrical Position/1 -> Theta/1
  IIR Filter/1 -> Speed_PU/1
  rad to PU_Pos/1 -> Speed Measurement/1, Mechanical to Electrical Position/1  "Pos_PU"
  rad/s to PU_Speed/1 -> Terminator1/1
